simulink model "lab09_2"  (R2014a)
settings: Solver=ode45  StartTime=0.0  StopTime=40  RelTol=1e-3
libraries: dsparch4 x1, commrandsrc2 x1, dspsrcs4 x1
settings Model: Creator=郑祖闯  LastModifiedBy=郑祖闯

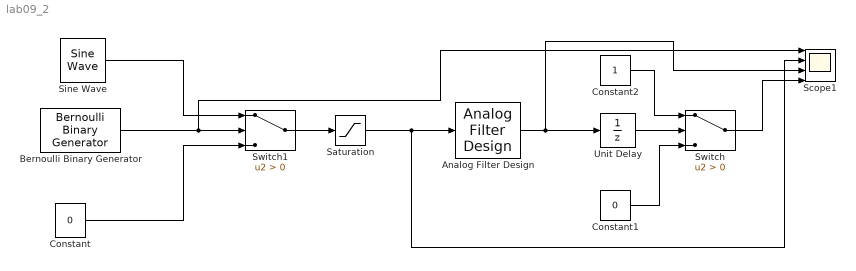
== system lab09_2 ==
  Analog Filter Design : dsparch4/Analog Filter Design  method=Butterworth  filttype=Lowpass  N=8  Wlo=4*pi  Whi=80  Rp=2  Rs=40
  Bernoulli Binary Generator : commrandsrc2/Bernoulli Binary Generator  P=0.5  seed=61  Ts=1  frameBased=off  sampPerFrame=1  orient=off  outDataType=double
  Constant : Constant  Value=0  VectorParams1D=off
  Constant1 : Constant  Value=0
  Constant2 : Constant
  Saturation : Saturate  UpperLimit=inf  LowerLimit=0
  Scope1 : Scope  NumInputPorts=4
      settings: TimeRange=40  YMin=-2~-1~-1~-2  YMax=2~1~1~2  SampleInput=on
  Sine Wave : dspsrcs4/Sine Wave  Amplitude=1  Frequency=2  Phase=0  SampleMode=Discrete  OutComplex=Real  CompMethod=Trigonometric fcn  TableSize=Speed  SampleTime=1/50  SamplesPerFrame=1  ResetState=Restart at time zero  dataType=double  wordLen=16  udDataType=sfix(16)  fracBitsMode=Best precision  numFracBits=15  OutDataTypeStr=double  LastOutDataTypeStr=double
  Switch : Switch  Criteria=u2 > Threshold
  Switch1 : Switch  Criteria=u2 > Threshold
  Unit Delay : UnitDelay
  wires:
  Bernoulli Binary Generator/1 -> Scope1/1, Switch1/2
  Sine Wave/1 -> Switch1/1
  Constant/1 -> Switch1/3
  Switch1/1 -> Saturation/1
  Saturation/1 -> Scope1/2, Analog Filter Design/1
  Analog Filter Design/1 -> Unit Delay/1, Scope1/3
  Switch/1 -> Scope1/4
  Constant1/1 -> Switch/3
  Constant2/1 -> Switch/1
  Unit Delay/1 -> Switch/2
